simulink model "Simulink1"  (R2017b)
settings: Solver=VariableStepAuto  StartTime=0.0  StopTime=100.0  RelTol=1e-3
libraries: simulink x6
settings Model: Creator=Mare  LastModifiedBy=Mare

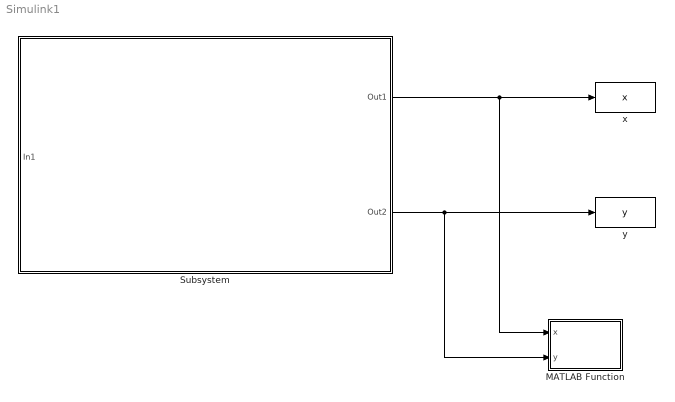
== system Simulink1 ==
  MATLAB Function : MATLAB Function  TreatAsAtomicUnit=on
  Subsystem : Subsystem
  x : ToWorkspace  VariableName=x  SaveFormat=Structure With Time  SampleTime=0.5
  y : ToWorkspace  VariableName=y  SaveFormat=Structure With Time  SampleTime=0.5
  wires:
  Subsystem/1(Out1) -> MATLAB Function/1(x), x/1
  Subsystem/2(Out2) -> MATLAB Function/2(y), y/1

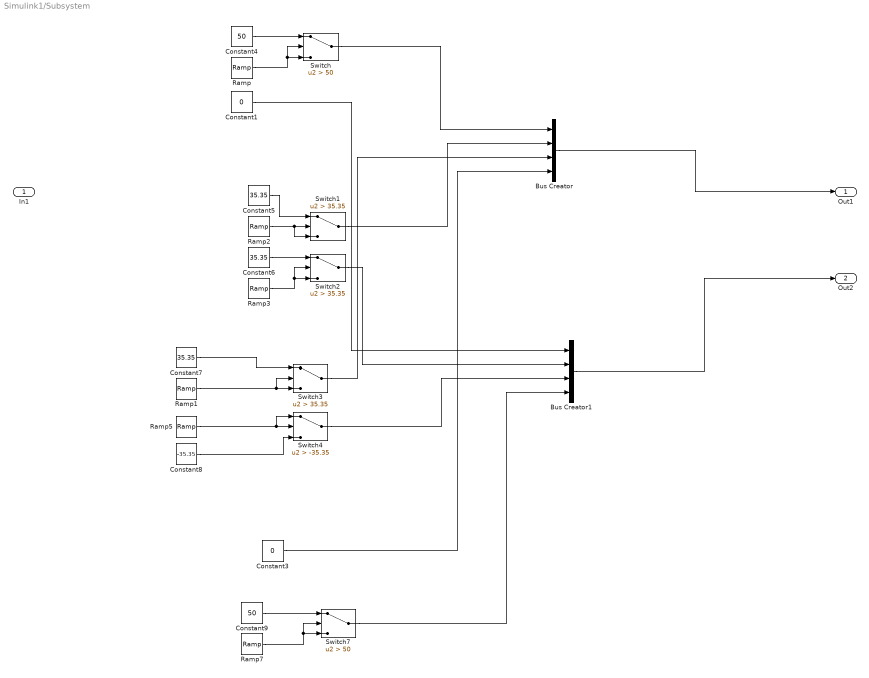
== system Simulink1/Subsystem ==
  In1 : Inport
  Bus Creator : BusCreator  Inputs=4
  Bus Creator1 : BusCreator  Inputs=4
  Constant1 : Constant  Value=0
  Constant3 : Constant  Value=0
  Constant4 : Constant  Value=50
  Constant5 : Constant  Value=35.35
  Constant6 : Constant  Value=35.35
  Constant7 : Constant  Value=35.35
  Constant8 : Constant  Value=-35.35
  Constant9 : Constant  Value=50
  Ramp{,1..3,7} (5 alike) : simulink/Sources/Ramp  slope=1  start=0  X0=0
  Ramp5 : simulink/Sources/Ramp  slope=-1  start=0  X0=0
  Switch : Switch  Criteria=u2 > Threshold  Threshold=50
  Switch1 : Switch  Criteria=u2 > Threshold  Threshold=35.35
  Switch2 : Switch  Criteria=u2 > Threshold  Threshold=35.35
  Switch3 : Switch  Criteria=u2 > Threshold  Threshold=35.35
  Switch4 : Switch  Criteria=u2 > Threshold  Threshold=-35.35
  Switch7 : Switch  Criteria=u2 > Threshold  Threshold=50
  Out1 : Outport
  Out2 : Outport  Port=2
  wires:
  Switch/1 -> Bus Creator/1
  Switch1/1 -> Bus Creator/2
  Bus Creator/1 -> Out1/1
  Constant1/1 -> Bus Creator1/1
  Switch2/1 -> Bus Creator1/2
  Bus Creator1/1 -> Out2/1
  Constant4/1 -> Switch/1
  Ramp/1 -> Switch/2, Switch/3
  Ramp2/1 -> Switch1/3, Switch1/2
  Constant5/1 -> Switch1/1
  Ramp3/1 -> Switch2/2, Switch2/3
  Constant6/1 -> Switch2/1
  Constant7/1 -> Switch3/1
  Constant8/1 -> Switch4/3
  Ramp1/1 -> Switch3/2, Switch3/3
  Ramp5/1 -> Switch4/1, Switch4/2
  Switch3/1 -> Bus Creator/3
  Switch4/1 -> Bus Creator1/3
  Ramp7/1 -> Switch7/2, Switch7/3
  Constant3/1 -> Bus Creator/4
  Constant9/1 -> Switch7/1
  Switch7/1 -> Bus Creator1/4

== matlab function Simulink1/MATLAB Function ==
  data: x input; y input
function  fcn(x,y)
%postavljanje granicnih vrijednosti koordinata
xmax = 100;
xmin = -100;
ymax = 100;
ymin = -100;

colors = {[0.6,0.9,0.6],[0,0.7,1],[0.85, 0.6,0.85],[1,0.8,0],[0.9,0.6,0.5]};


cla;
axis([xmin,xmax,ymin,ymax]);
xlabel('x');
ylabel('y');
grid on;

for k = 1:length(x)
    plot(x(k),y(k),'o', 'Color', colors{k});
    hold on;
end

coder.extrinsic('legend');
legend('a1', 'a2', 'a3', 'a4');
